simulink model "Pacemaker"  (R2024b)
settings: Solver=FixedStepAuto  StartTime=0.0  StopTime=10  FixedStep=1e-3  RelTol=1e-3  EnableMultiTasking=on
undefined symbols (not defined in the file): D10, D11, D12, D2, D3, D4, D7, D8, D9, PTA0, PTA1, PTB23, PTB9, PTC3, PTC4, PTD0, PTD2, PTD3
libraries: frdmk64flib x9
settings Model: ExtModeTrigDuration=5  Creator=ltgoa  LastModifiedBy=ltgoa
settings OptimizationCC: DefaultParameterBehavior=Inlined  EnhancedBackFolding=on  PassReuseOutputArgsAs=Individual arguments  ZeroExternalMemoryAtStartup=off  ZeroInternalMemoryAtStartup=off  MaxStackSize=64  OptimizeBlockOrder=speed  DifferentSizesBufferReuse=on  OptimizationCustomize=off  EfficientTunableParamExpr=on
settings DebuggingCC: ParameterTunabilityLossMsg=error
settings HardwareCC: ProdBitPerPointer=32  ProdBitPerSizeT=32  ProdBitPerPtrDiffT=32  ProdLargestAtomicInteger=Long  ProdLargestAtomicFloat=Double  ProdWordSize=32  ProdHWDeviceType=ARM Compatible->ARM Cortex
settings SFSimCC: MATLABDynamicMemAlloc=off
settings RTWCC: Description=Embedded Coder  SystemTargetFile=ert.tlc  HardwareBoard=NXP FRDM-K64F  TLCOptions="-aInlineSetEventsForThisBaseRateFcn=TLC_FALSE -aSuppressMultiTaskScheduler=TLC_FALSE  -aRateBasedStepFcn=0"  TemplateMakefile=ert_default_tmf  Toolchain=GNU Tools for ARM Embedded Processors
settings CodeAppCC: ForceParamTrailComments=on  IgnoreCustomStorageClasses=off  OperatorAnnotations=on  SimulinkDataObjDesc=on  SFDataObjDesc=on  InsertBlockDesc=on
settings ERTTargetCC: ExtModeTransport=4  ExtModeMexFile=sendToCommService

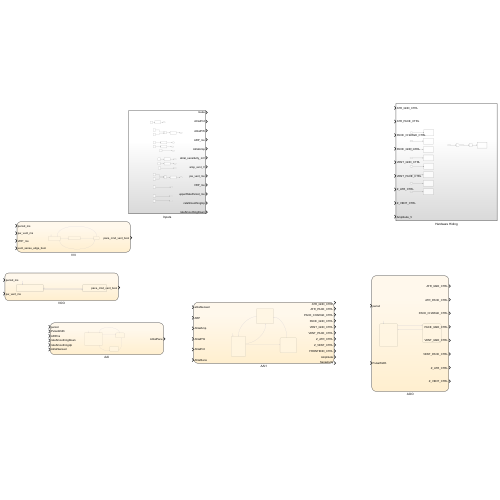
[thumbnail: Simulink's stored preview of the top-level diagram]
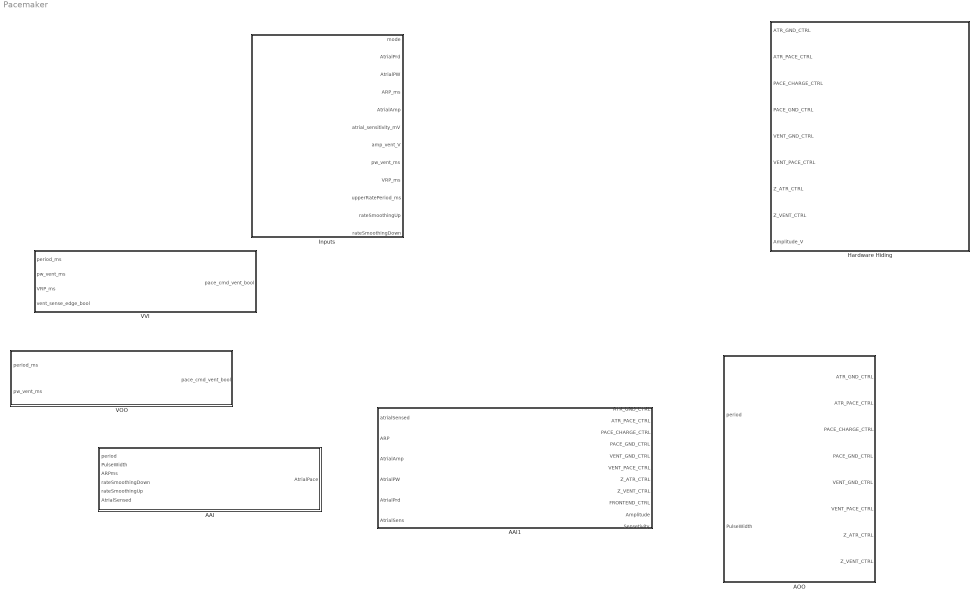
== system Pacemaker ==
  AAI : Stateflow chart  TreatAsAtomicUnit=on
      settings: PortSchema="{\"entries\":[{\"content\":{\"sides\":[{\"content\":{\"connectorIds\":[\"In1\",\"In2\",\"In4\",\"In5\",\"In6\",\"In3\"]},\"type\":\"ConnectorPlacement.EquallySpacedRectSide\",\"uuid\":\"973661e6-4611-4c0a-87fe-406229ab40c7\"},{\"content\":{\"connectorIds\":[\"Out1\"],\"side\":\"RIGHT\"},\"type\":\"ConnectorPlacement.EquallySpacedRectSide\",\"uuid\":\"cdcd0c3e-bb96-4d1d-a592-5b3edd861415\"},{\"content\":{\"side\":\"TOP\"},\"type\":\"ConnectorPlacement.EquallySpacedRectSide\",\"uuid\":\"ad33bfd1-9008-43d1-83e4-0c4f03eb0ba9\"}]},\"type\":\"ConnectorPlacement.EquallySpacedConnector\",\"uuid\":\"fdc4c0e3-7319-4af3-a318-dce7ba47455b\"}],\"packageUris\":[\"http://schema.mathworks.com/mf0/Connector/R2020b\"],\"version\":\"1.0\"}"
  AAI1 : Stateflow chart  TreatAsAtomicUnit=on
  AOO : Stateflow chart  TreatAsAtomicUnit=on
  Hardware Hiding : Subsystem
  Inputs : Subsystem
  VOO : Stateflow chart  TreatAsAtomicUnit=on
  VVI : Stateflow chart  TreatAsAtomicUnit=on
      settings: PortSchema="{\"entries\":[{\"content\":{\"sides\":[{\"content\":{\"connectorIds\":[\"In3\",\"In1\",\"In2\",\"In4\"]},\"type\":\"ConnectorPlacement.EquallySpacedRectSide\",\"uuid\":\"2814cae3-bb69-4b6f-8093-55c6c370e3d7\"},{\"content\":{\"connectorIds\":[\"Out1\"],\"side\":\"RIGHT\"},\"type\":\"ConnectorPlacement.EquallySpacedRectSide\",\"uuid\":\"4bf90426-a7eb-417e-ae62-88cacffde5ae\"},{\"content\":{\"side\":\"TOP\"},\"type\":\"ConnectorPlacement.EquallySpacedRectSide\",\"uuid\":\"76e9ef85-2922-4565-afc0-ab7cf3c2bb27\"}]},\"type\":\"ConnectorPlacement.EquallySpacedConnector\",\"uuid\":\"ba9b0447-7ffb-4daf-9277-ed94c76b7817\"}],\"packageUris\":[\"http://schema.mathworks.com/mf0/Connector/R2020b\"],\"version\":\"1.0\"}"

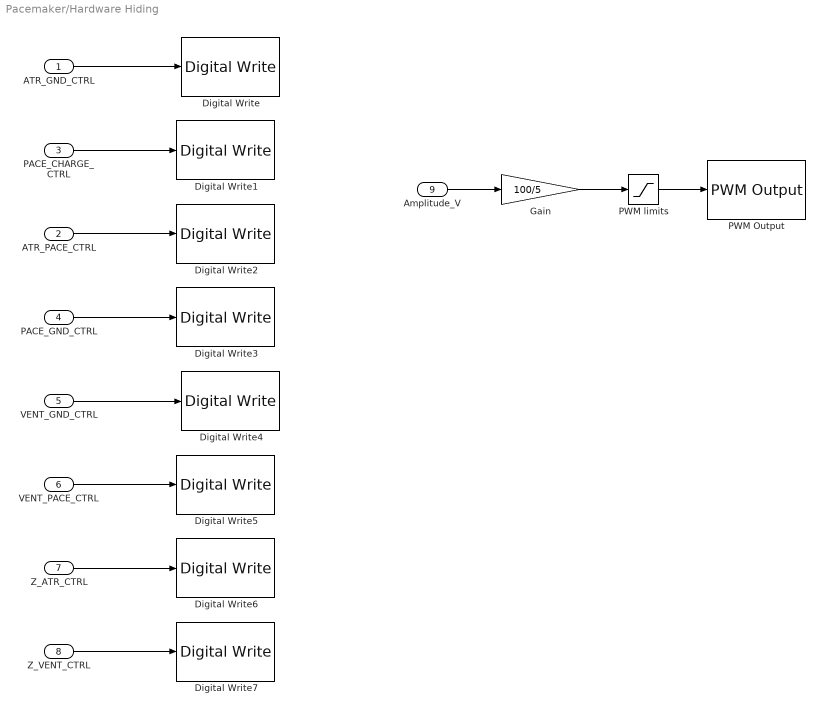
== system Pacemaker/Hardware Hiding ==
  ATR_GND_CTRL : Inport
  ATR_PACE_CTRL : Inport  Port=2
  PACE_CHARGE_CTRL : Inport  Port=3
  PACE_GND_CTRL : Inport  Port=4
  VENT_GND_CTRL : Inport  Port=5
  VENT_PACE_CTRL : Inport  Port=6
  Z_ATR_CTRL : Inport  Port=7
  Z_VENT_CTRL : Inport  Port=8
  Amplitude_V : Inport  Port=9
  Digital Write : frdmk64flib/Digital Write  Whichpin=PTD2 (D11)
  Digital Write1 : frdmk64flib/Digital Write  Whichpin=PTB9 (D2)
  Digital Write2 : frdmk64flib/Digital Write  Whichpin=PTA0 (D8)
  Digital Write3 : frdmk64flib/Digital Write  Whichpin=PTD0 (D10)
  Digital Write4 : frdmk64flib/Digital Write  Whichpin=PTD3 (D12)
  Digital Write5 : frdmk64flib/Digital Write  Whichpin=PTC4 (D9)
  Digital Write6 : frdmk64flib/Digital Write  Whichpin=PTB23 (D4)
  Digital Write7 : frdmk64flib/Digital Write  Whichpin=PTC3 (D7)
  Gain : Gain  Gain=100/5
  PWM Output : frdmk64flib/PWM Output  Whichpin=PTA1 (D3)  InitialFrequency=2000  InitialDutyCycle=0
  PWM limits : Saturate  UpperLimit=100  LowerLimit=0
  wires:
  ATR_GND_CTRL/1 -> Digital Write/1
  PACE_CHARGE_CTRL/1 -> Digital Write1/1
  ATR_PACE_CTRL/1 -> Digital Write2/1
  PACE_GND_CTRL/1 -> Digital Write3/1
  VENT_GND_CTRL/1 -> Digital Write4/1
  VENT_PACE_CTRL/1 -> Digital Write5/1
  Z_ATR_CTRL/1 -> Digital Write6/1
  Z_VENT_CTRL/1 -> Digital Write7/1
  Amplitude_V/1 -> Gain/1
  Gain/1 -> PWM limits/1
  PWM limits/1 -> PWM Output/1

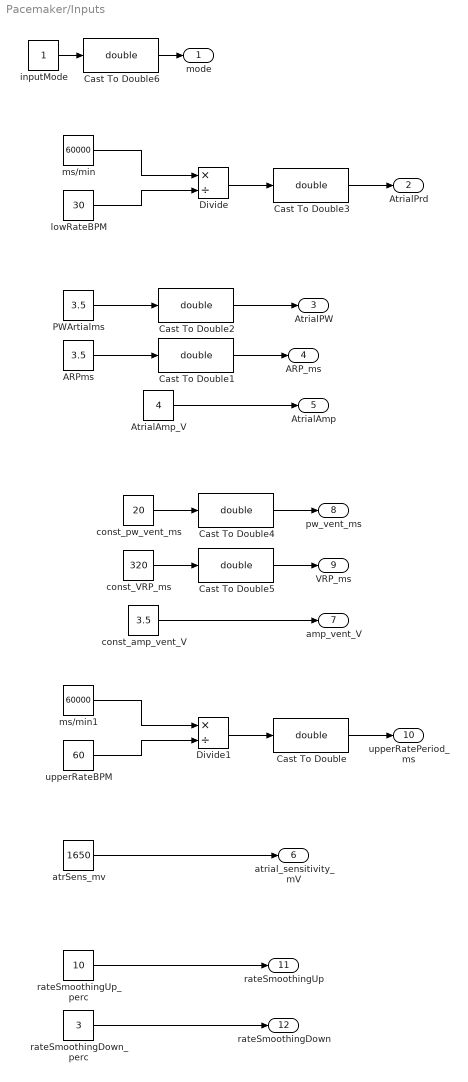
== system Pacemaker/Inputs ==
  ARPms : Constant  Value=3.5
  AtrialAmp_V : Constant  Value=4
  Cast To Double{,1..6} (7 alike) : DataTypeConversion  OutDataTypeStr=double  SaturateOnIntegerOverflow=off  RndMeth=Floor
  Divide : Product  Inputs=*/
  Divide1 : Product  Inputs=*/
  PWArtialms : Constant  Value=3.5
  atrSens_mv : Constant  Value=1650
  const_VRP_ms : Constant  Value=320
  const_amp_vent_V : Constant  Value=3.5
  const_pw_vent_ms : Constant  Value=20
  inputMode : Constant
  lowRateBPM : Constant  Value=30
  ms/min : Constant  Value=60000
  ms/min1 : Constant  Value=60000
  rateSmoothingDown_perc : Constant  Value=3
  rateSmoothingUp_perc : Constant  Value=10
  upperRateBPM : Constant  Value=60
  mode : Outport
  AtrialPrd : Outport  Port=2
  AtrialPW : Outport  Port=3
  ARP_ms : Outport  Port=4
  AtrialAmp : Outport  Port=5
  atrial_sensitivity_mV : Outport  Port=6
  amp_vent_V : Outport  Port=7
  pw_vent_ms : Outport  Port=8
  VRP_ms : Outport  Port=9
  upperRatePeriod_ms : Outport  Port=10
  rateSmoothingUp : Outport  Port=11
  rateSmoothingDown : Outport  Port=12
  wires:
  AtrialAmp_V/1 -> AtrialAmp/1
  PWArtialms/1 -> Cast To Double2/1
  ms/min/1 -> Divide/1
  lowRateBPM/1 -> Divide/2
  Divide/1 -> Cast To Double3/1
  Cast To Double3/1 -> AtrialPrd/1
  Cast To Double2/1 -> AtrialPW/1
  Cast To Double5/1 -> VRP_ms/1
  const_VRP_ms/1 -> Cast To Double5/1
  const_pw_vent_ms/1 -> Cast To Double4/1
  Cast To Double4/1 -> pw_vent_ms/1
  const_amp_vent_V/1 -> amp_vent_V/1
  upperRateBPM/1 -> Divide1/2
  Divide1/1 -> Cast To Double/1
  ms/min1/1 -> Divide1/1
  atrSens_mv/1 -> atrial_sensitivity_mV/1
  rateSmoothingUp_perc/1 -> rateSmoothingUp/1
  rateSmoothingDown_perc/1 -> rateSmoothingDown/1
  Cast To Double/1 -> upperRatePeriod_ms/1
  ARPms/1 -> Cast To Double1/1
  Cast To Double1/1 -> ARP_ms/1
  inputMode/1 -> Cast To Double6/1
  Cast To Double6/1 -> mode/1

== stateflow chart Pacemaker/AAI1 ==
  state ARP_STATE
    entry:
    %Charge C22
    PACE_CHARGE_CTRL = true;
    ATR_PACE_CTRL = false;
    VENT_PACE_CTRL = false;
    %Discharge C21
    PACE_GND_CTRL = true;
    Z_ATR_CTRL = false;
    Z_VENT_CTRL = false;
    ATR_GND_CTRL = true;
    VENT_GND_CTRL = false;
    %Turn on sensing logic
    FRONTEND_CTRL=true;
  state WAIT_CHARGE
    entry:
    %Set variables
    Amplitude = AtrialAmp;
    period = AtrialPrd;
    PulseWidth = AtrialPW;
    Sensetivity = AtrialSens;
    %Charge C22
    PACE_CHARGE_CTRL = true;
    ATR_PACE_CTRL = false;
    VENT_PACE_CTRL = false;
    %Discharge C21
    PACE_GND_CTRL = true;
    Z_ATR_CTRL = false;
    Z_VENT_CTRL = false;
    ATR_GND_CTRL = true;
    VENT_GND_CTRL = false;
    %Turn on sensing logic
    FRONTEND_CTRL=true;
  state PACE_DISCHARGE
    entry:
    %Pace atrial valve
    PACE_CHARGE_CTRL = false;
    PACE_GND_CTRL = true;
    ATR_PACE_CTRL = true;
    ATR_GND_CTRL = false;
    Z_ATR_CTRL = false;
    Z_VENT_CTRL = false;
    VENT_GND_CTRL = false;
    VENT_PACE_CTRL = false;
    %Disable sensing logic during pulse
    FRONTEND_CTRL = false;
  ARP_STATE -> WAIT_CHARGE : [after(ARP, msec)]
  PACE_DISCHARGE -> ARP_STATE : [after(PulseWidth, msec)]
  WAIT_CHARGE -> ARP_STATE [order 2] : [atrialSensed == true]
  (default) -> WAIT_CHARGE
  WAIT_CHARGE -> PACE_DISCHARGE [order 1] : [after(period-PulseWidth, msec)]
  data: ATR_GND_CTRL output boolean size=1; ATR_PACE_CTRL output boolean size=1; PACE_CHARGE_CTRL output boolean size=1; PACE_GND_CTRL output boolean size=1; VENT_GND_CTRL output boolean size=1; VENT_PACE_CTRL output boolean size=1; Z_ATR_CTRL output boolean size=1; Z_VENT_CTRL output boolean size=1; FRONTEND_CTRL output boolean size=1; atrialSensed input boolean size=1; ARP input double size=1; period local double size=1; AtrialAmp input double size=1; AtrialPW input double size=1; AtrialPrd input double size=1; Amplitude output double size=1; PulseWidth local double size=1; AtrialSens input double size=1; Sensetivity output double size=1

== stateflow chart Pacemaker/AAI ==
  state WAIT
    entry:
    AtrialPace = false;
    %rate smoothing
    minRate = prevPeriod * (1-rateSmoothingUp/100);
    maxRate = prevPeriod * (1+rateSmoothingDown/100);
    if(period < minRate)
    smoothed_period = minRate;
    elseif (period > maxRate)
    smoothed_period = maxRate;
    else
    smoothed_period = period;
    end
    prevPeriod = smoothed_period;
  state ARP
    entry:
    AtrialPace = false;
  state PACE
    entry:
    AtrialPace = true;
  ARP -> WAIT : [after(ARPms, msec)]
  (default) -> WAIT
  WAIT -> ARP [order 2] : [AtrialSensed==true]
  PACE -> ARP : [after(PulseWidth, msec)]
  WAIT -> PACE [order 1] : [after(smoothed_period, msec)]
  data: period input double; PulseWidth input double; AtrialPace output boolean; AtrialSensed input boolean; ARPms input double; prevPeriod local double =100; maxRate local double; minRate local double; smoothed_period local double; rateSmoothingDown input double; rateSmoothingUp input double

== stateflow chart Pacemaker/VOO ==
  state WAIT
    entry:
    pace_cmd_vent_bool = false;
  state PACE
    entry:
    pace_cmd_vent_bool = true;
  (default) -> WAIT
  PACE -> WAIT : after(pw_vent_ms, msec)
  WAIT -> PACE : after(period_ms - pw_vent_ms, msec)
  data: period_ms input; pw_vent_ms input; pace_cmd_vent_bool output boolean

== stateflow chart Pacemaker/VVI ==
  state WAIT
    entry: pace_cmd_vent_bool = false;
  state PACE
    entry: pace_cmd_vent_bool = true;
    exit: pace_cmd_vent_bool = false;
  state VRP
  VRP -> WAIT : [after(VRP_ms, msec)]
  (default) -> WAIT
  WAIT -> PACE [order 1] : [after(period_ms, msec)]
  PACE -> VRP : [after(pw_vent_ms, msec)]
  WAIT -> VRP [order 2] : [vent_sense_edge_bool]
  data: pw_vent_ms input double; VRP_ms input; period_ms input; pace_cmd_vent_bool output boolean; vent_sense_edge_bool input boolean

== stateflow chart Pacemaker/AOO ==
  state WAIT_CHARGE
    entry:
    %Charge C22
    PACE_CHARGE_CTRL = true;
    ATR_PACE_CTRL = false;
    VENT_PACE_CTRL = false;
    %Discharge C21
    PACE_GND_CTRL = true;
    Z_ATR_CTRL = false;
    Z_VENT_CTRL = false;
    ATR_GND_CTRL = true;
    VENT_GND_CTRL = false;
  state PACE_ATRIAL
    entry:
    %Pace atrial valve
    PACE_CHARGE_CTRL = false;
    PACE_GND_CTRL = true;
    ATR_PACE_CTRL = true;
    ATR_GND_CTRL = false;
    Z_ATR_CTRL = false;
    Z_VENT_CTRL = false;
    VENT_GND_CTRL = false;
    VENT_PACE_CTRL = false;
  (default) -> WAIT_CHARGE
  WAIT_CHARGE -> PACE_ATRIAL : [after(period - PulseWidth, msec)]
  PACE_ATRIAL -> WAIT_CHARGE : [after(PulseWidth, msec)]
  data: ATR_GND_CTRL output; ATR_PACE_CTRL output; PACE_CHARGE_CTRL output; PACE_GND_CTRL output; VENT_GND_CTRL output; VENT_PACE_CTRL output; Z_ATR_CTRL output; Z_VENT_CTRL output; period input; PulseWidth input
